simulink model "PH1_uGrid_ZC_carga"  (R2017a)
settings: Solver=ode4  StartTime=0.0  StopTime=6  FixedStep=1e-6  MaxStep=1e-4  RelTol=1e-3
InitFcn:
  | SimulinkInit
values from neighbouring files (symbols this model uses):
  J = 0.3    [SimulinkInit.m]
  K1 = 1.15    [SimulinkInit.m]
  K2 = 1    [SimulinkInit.m]
  K3 = 1    [SimulinkInit.m]
  P = 0.1    [SimulinkInit.m]
  Tao1 = 0.5    [SimulinkInit.m]
  Tao2 = 0.125    [SimulinkInit.m]
undefined symbols (not defined in the file or in its folder): G, GF, Ion, Lithium
libraries: powerlib x58, dsparch4 x12, powerlib_meascontrol x5, fl_lib x5, nesl_utility x4, mpclib x2, electricdrivelib x1, simulink x1
(part 2 of 2)

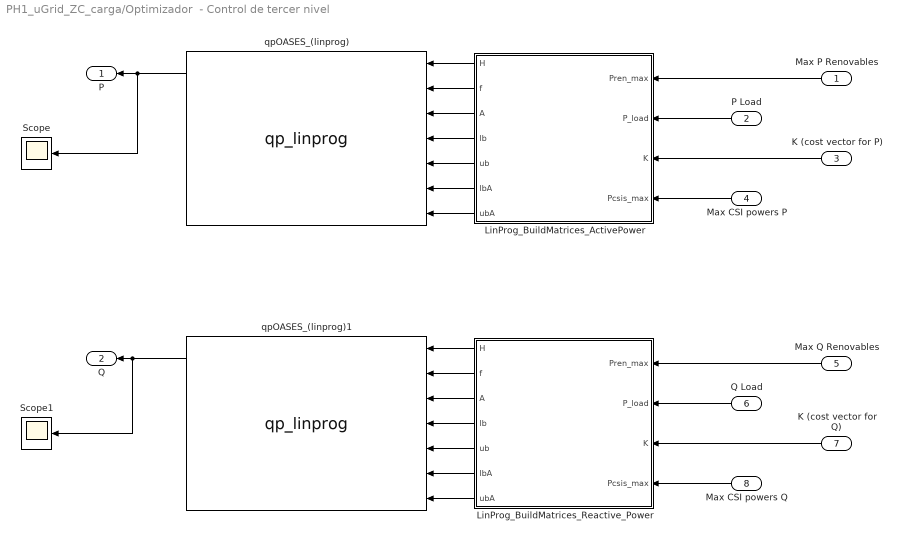
== system PH1_uGrid_ZC_carga/Optimizador  - Control de tercer nivel ==
  Max P Renovables : Inport
  P Load : Inport  Port=2
  K (cost vector for P) : Inport  Port=3
  Max CSI powers P : Inport  Port=4
  Max Q Renovables : Inport  Port=5
  Q Load : Inport  Port=6
  K (cost vector for Q) : Inport  Port=7
  Max CSI powers Q : Inport  Port=8
  LinProg_BuildMatrices_ActivePower : MATLAB Function  TreatAsAtomicUnit=on
  LinProg_BuildMatrices_Reactive_Power : MATLAB Function  TreatAsAtomicUnit=on
  Scope : Scope
  Scope1 : Scope
  qpOASES_(linprog) : S-Function  FunctionName=qp_linprog  SFunctionDeploymentMode=off  EnableBusSupport=off
  qpOASES_(linprog)1 : S-Function  FunctionName=qp_linprog  SFunctionDeploymentMode=off  EnableBusSupport=off
  P : Outport
  Q : Outport  Port=2
  wires:
  Max CSI powers P/1 -> LinProg_BuildMatrices_ActivePower/4(Pcsis_max)
  Max P Renovables/1 -> LinProg_BuildMatrices_ActivePower/1(Pren_max)
  LinProg_BuildMatrices_ActivePower/6(lbA) -> qpOASES_(linprog)/6
  LinProg_BuildMatrices_ActivePower/5(ub) -> qpOASES_(linprog)/5
  LinProg_BuildMatrices_ActivePower/7(ubA) -> qpOASES_(linprog)/7
  LinProg_BuildMatrices_ActivePower/2(f) -> qpOASES_(linprog)/2
  LinProg_BuildMatrices_ActivePower/4(lb) -> qpOASES_(linprog)/4
  LinProg_BuildMatrices_ActivePower/1(H) -> qpOASES_(linprog)/1
  K (cost vector for P)/1 -> LinProg_BuildMatrices_ActivePower/3(K)
  P Load/1 -> LinProg_BuildMatrices_ActivePower/2(P_load)
  LinProg_BuildMatrices_ActivePower/3(A) -> qpOASES_(linprog)/3
  LinProg_BuildMatrices_Reactive_Power/1(H) -> qpOASES_(linprog)1/1
  LinProg_BuildMatrices_Reactive_Power/5(ub) -> qpOASES_(linprog)1/5
  LinProg_BuildMatrices_Reactive_Power/3(A) -> qpOASES_(linprog)1/3
  LinProg_BuildMatrices_Reactive_Power/4(lb) -> qpOASES_(linprog)1/4
  LinProg_BuildMatrices_Reactive_Power/6(lbA) -> qpOASES_(linprog)1/6
  LinProg_BuildMatrices_Reactive_Power/2(f) -> qpOASES_(linprog)1/2
  LinProg_BuildMatrices_Reactive_Power/7(ubA) -> qpOASES_(linprog)1/7
  qpOASES_(linprog)/1 -> Scope/1, P/1
  qpOASES_(linprog)1/1 -> Scope1/1, Q/1
  Q Load/1 -> LinProg_BuildMatrices_Reactive_Power/2(P_load)
  K (cost vector for Q)/1 -> LinProg_BuildMatrices_Reactive_Power/3(K)
  Max Q Renovables/1 -> LinProg_BuildMatrices_Reactive_Power/1(Pren_max)
  Max CSI powers Q/1 -> LinProg_BuildMatrices_Reactive_Power/4(Pcsis_max)

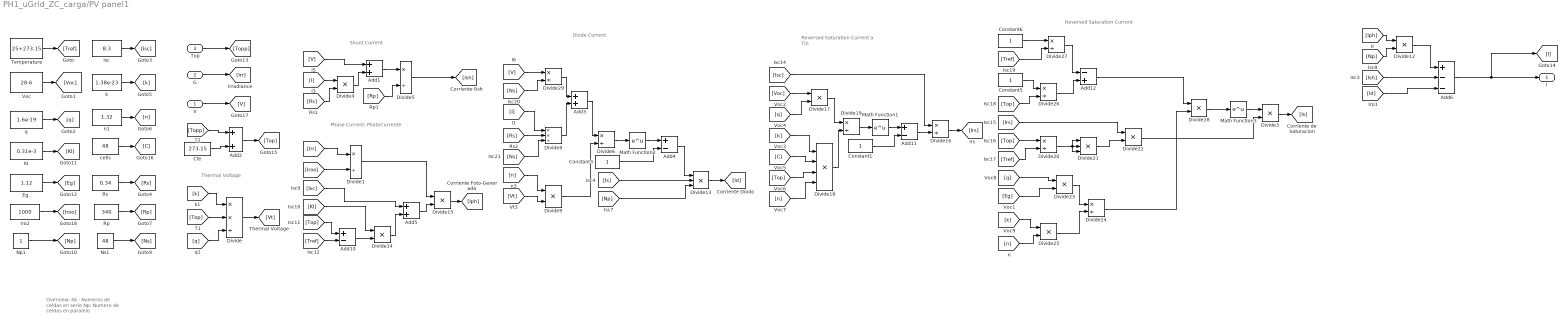
== system PH1_uGrid_ZC_carga/PV panel1 ==
  note: Overview:
      | Ns : Numeros de celdas en serie
      | Np: Numero de celdas en paralelo
  note: Thermal Voltage
  note: Shunt Current
  note: Phase Current- PhotoCurrente
  note: Diode Current
  note: Reversed Saturation Current a Tin
  note: Reversed Saturation Current
  V : Inport
  G : Inport  Port=2
  Top : Inport  Port=3
  Add{1..3,5} (4 alike) : Sum
  Add10 : Sum  Inputs=+-
  Add11 : Sum  Inputs=+-
  Add12 : Sum  Inputs=-+
  Add4 : Sum  Inputs=+-
  Add6 : Sum  Inputs=+--
  Constant{1,3,5..6} (4 alike) : Constant
  Cte : Constant  Value=273.15
  Divide : Product  Inputs=**/
  Divide{1,5..6,16,19..20,24,26..27,29} (10 alike) : Product  Inputs=*/
  Divide{3..4,9,12,14..15,17,22..23,25,28} (11 alike) : Product  Inputs=**
  Divide13 : Product  Inputs=***
  Divide18 : Product  Inputs=****
  Divide21 : Product  Inputs=***
  Divide8 : Product  Inputs=**/
  Eg. : Constant  Value=1.12
  Iro2 : Constant  Value=1000
  Isc : Constant  Value=8.3
  KI : Constant  Value=0.31e-3
  Math Function1 : Math  SaturateOnIntegerOverflow=on
  Math Function2 : Math  SaturateOnIntegerOverflow=on
  Math Function3 : Math  SaturateOnIntegerOverflow=on
  Np1 : Constant
  Ns1 : Constant  Value=48
  Rp : Constant  Value=340
  Rs : Constant  Value=0.34
  Temperature : Constant  Value=25+273.15
  Voc : Constant  Value=28.6
  cells : Constant  Value=48
  k : Constant  Value=1.38e-23
  n1 : Constant  Value=1.32
  q : Constant  Value=1.6e-19
  I : Outport
  wires:
  Temperature/1 -> [Tref]
  Voc/1 -> [Voc]
  q/1 -> [q]
  Isc/1 -> [Isc]
  k/1 -> [k]
  n1/1 -> [n]
  [k] -> Divide/1
  [Top] -> Divide/2
  [q] -> Divide/3
  Divide/1 -> [Vt]
  Divide3/1 -> [Is]
  [Ish] -> Add6/2
  Add6/1 -> I/1, [I]
  [I] -> Divide8/1
  [Rs] -> Divide8/2
  Divide8/1 -> Add3/2
  [n] -> Divide9/1
  [Vt] -> Divide9/2
  Divide9/1 -> Divide6/2
  Add3/1 -> Divide6/1
  Divide6/1 -> Math Function2/1
  Math Function2/1 -> Add4/1
  Add4/1 -> Divide13/1
  [Is] -> Divide13/2
  Divide13/1 -> [Id]
  Divide4/1 -> Add1/2
  Add1/1 -> Divide5/1
  [Rp] -> Divide5/2
  Divide5/1 -> [Ish]
  [Rs] -> Divide4/2
  [I] -> Divide4/1
  KI/1 -> [KI]
  Eg./1 -> [Eg]
  [V] -> Add1/1
  [Np] -> Divide13/3
  [Iph] -> Divide12/1
  [Np] -> Divide12/2
  Divide12/1 -> Add6/1
  [Isc] -> Add5/1
  [Top] -> Add10/1
  [Tref] -> Add10/2
  Add10/1 -> Divide14/2
  [KI] -> Divide14/1
  [Voc] -> Divide17/1
  [q] -> Divide17/2
  [k] -> Divide18/1
  [C] -> Divide18/2
  [Top] -> Divide18/3
  [n] -> Divide18/4
  Divide17/1 -> Divide19/1
  Divide18/1 -> Divide19/2
  Divide19/1 -> Math Function1/1
  Constant1/1 -> Add11/2
  Math Function1/1 -> Add11/1
  Add11/1 -> Divide16/2
  Divide16/1 -> [Irs]
  [Tref] -> Divide20/2
  [Top] -> Divide20/1
  Divide20/1 -> Divide21/2, Divide21/1, Divide21/3
  Divide21/1 -> Divide22/2
  [Irs] -> Divide22/1
  [q] -> Divide23/1
  Divide23/1 -> Divide24/1
  [k] -> Divide25/1
  [n] -> Divide25/2
  Divide25/1 -> Divide24/2
  Constant5/1 -> Divide26/1
  [Top] -> Divide26/2
  Constant6/1 -> Divide27/1
  [Tref] -> Divide27/2
  Divide27/1 -> Add12/1
  Divide26/1 -> Add12/2
  Add12/1 -> Divide28/1
  Divide24/1 -> Divide28/2
  Divide28/1 -> Math Function3/1
  Divide29/1 -> Add3/1
  [Ns] -> Divide29/2
  [V] -> Divide29/1
  [Ns] -> Divide8/3
  Divide14/1 -> Add5/2
  Add5/1 -> Divide15/2
  Divide15/1 -> [Iph]
  V/1 -> [V]
  G/1 -> [Irr]
  Top/1 -> [Topp]
  cells/1 -> [C]
  [Id] -> Add6/3
  Cte/1 -> Add2/2
  Add2/1 -> [Top]
  [Topp] -> Add2/1
  [Irr] -> Divide1/1
  [Iroo] -> Divide1/2
  Divide1/1 -> Divide15/1
  Iro2/1 -> [Iroo]
  Rs/1 -> [Rs]
  Rp/1 -> [Rp]
  Ns1/1 -> [Ns]
  Np1/1 -> [Np]
  Constant3/1 -> Add4/2
  [Isc] -> Divide16/1
  Math Function3/1 -> Divide3/1
  Divide22/1 -> Divide3/2
  [Eg] -> Divide23/2

== system PH1_uGrid_ZC_carga/Subsystem ==
  In1 : Inport
  Controlled Current Source : fl_lib/Electrical/Electrical Sources/Controlled Current Source
  Current Sensor : fl_lib/Electrical/Electrical Sensors/Current Sensor
  Electrical Reference : fl_lib/Electrical/Electrical Elements/Electrical Reference
  Id1 : Display
  Id3 : Display
  PS-Simulink Converter : nesl_utility/PS-Simulink Converter  PhysicalDomain=network_engine_domain  SubClassName=ps_output  LeftPortType=input  RightPortType=output  PseudoPeriodic=off  Frequencies=[]  Unit=1  AffineConversion=off
  PS-Simulink Converter1 : nesl_utility/PS-Simulink Converter  PhysicalDomain=network_engine_domain  SubClassName=ps_output  LeftPortType=input  RightPortType=output  PseudoPeriodic=off  Frequencies=[]  Unit=1  AffineConversion=off
  Resistor : fl_lib/Electrical/Electrical Elements/Resistor  R=10.02 Ohm  i_specify=off  i_priority=High  i=0 A  i_nominal_specify=off  i_nominal_unit=A  i_nominal_value=1  v_specify=off  v_priority=High  v=0 V  v_nominal_specify=off  v_nominal_unit=V  v_nominal_value=1
  Simulink-PS Converter1 : nesl_utility/Simulink-PS Converter  PhysicalDomain=network_engine_domain  SubClassName=ps_input  LeftPortType=input  RightPortType=output  PseudoPeriodic=off  Frequencies=[]  NoiseDistribution=none  NoiseParameters=[]  Unit=1  AffineConversion=off  FilteringAndDerivatives=zero  SimscapeFilterOrder=1  InputFilterTimeConstant=.000001  UdotUserProvided=0
  Solver Configuration : nesl_utility/Solver Configuration  PhysicalDomain=network_engine_domain  SubClassName=solver  LeftPortType=input  RightPortType=generic  Accelerate=off  Tones=[]  Harmonics=[]  SimulateNoise=off  Profile=off  UseLocalSampling=off  EnableSwitchedLinearOptims=on  FrequencyDomain=off  UseCCode=off  RelTol=0.001  AbsTol=1e-06  MinStep=1e-09  ToWorkspace=off  RevertToSquareIcSolve=off  NumHomotopyIterations=100  PhasorMode=off  PhasorModeNumHarmonics=1  OverrideAbsTol=off  DoDC=on  ResidualTolerance=1e-8  UseLocalSolver=on  LocalSolverChoice=NE_BACKWARD_EULER_ADVANCER  LocalSolverSampleTime=.1  DoFixedCost=off  MaxNonlinIter=8  MaxModeIter=2  LinearAlgebra=Sparse  DelaysMemoryBudget=1024  AutomaticFiltering=on  FilteringTimeConstant=0.001
  Voltage Sensor : fl_lib/Electrical/Electrical Sensors/Voltage Sensor
  V1 : Outport
  I : Outport  Port=2
  wires:
  PS-Simulink Converter1/1 -> I/1, Id1/1
  PS-Simulink Converter/1 -> V1/1, Id3/1
  In1/1 -> Simulink-PS Converter1/1
  connections:
  Voltage Sensor/RConn1 -- PS-Simulink Converter/LConn1
  Current Sensor/RConn2 -- Voltage Sensor/LConn1 -- Resistor/LConn1
  Controlled Current Source/RConn1 -- Simulink-PS Converter1/RConn1
  Electrical Reference/LConn1 -- Voltage Sensor/RConn2 -- Resistor/RConn1 -- Controlled Current Source/RConn2
  Current Sensor/RConn1 -- PS-Simulink Converter1/LConn1
  Controlled Current Source/LConn1 -- Current Sensor/LConn1 -- Solver Configuration/RConn1

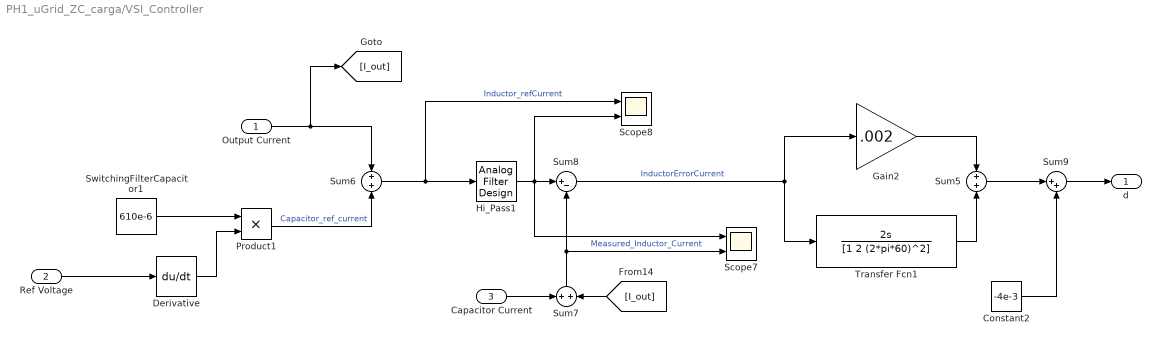
== system PH1_uGrid_ZC_carga/VSI_Controller ==
  Output Current : Inport
  Ref Voltage : Inport  Port=2
  Capacitor Current : Inport  Port=3
  Constant2 : Constant  Value=-4e-3
  Derivative : Derivative  CoefficientInTFapproximation=1e-3
  Gain2 : Gain  Gain=.002
  Hi_Pass1 : dsparch4/Analog Filter Design  method=Bessel  filttype=Highpass  N=1  Wlo=1*2*pi  Whi=80  Rp=2  Rs=40
  Product1 : Product
  Scope7 : Scope  NumInputPorts=2
  Scope8 : Scope  NumInputPorts=2
  Sum5 : Sum  Inputs=+|+
  Sum6 : Sum  Inputs=+|+
  Sum7 : Sum  Inputs=+|+
  Sum8 : Sum  Inputs=|+-
  Sum9 : Sum  Inputs=|++
  SwitchingFilterCapacitor1 : Constant  Value=610e-6
  Transfer Fcn1 : TransferFcn  Numerator=[2 0]  Denominator=[1 2 (2*pi*60)^2]
  d : Outport
  wires:
  Derivative/1 -> Product1/2
  Sum6/1 -> Hi_Pass1/1, Scope8/1  "Inductor_refCurrent"
  Sum8/1 -> Transfer Fcn1/1, Gain2/1  "InductorErrorCurrent"
  Ref Voltage/1 -> Derivative/1
  Constant2/1 -> Sum9/2
  Capacitor Current/1 -> Sum7/1
  Transfer Fcn1/1 -> Sum5/2
  Output Current/1 -> Sum6/1, [I_out]
  [I_out] -> Sum7/2
  Gain2/1 -> Sum5/1
  SwitchingFilterCapacitor1/1 -> Product1/1
  Hi_Pass1/1 -> Scope8/2, Sum8/1, Scope7/1
  Product1/1 -> Sum6/2  "Capacitor_ref_current"
  Sum9/1 -> d/1
  Sum5/1 -> Sum9/1
  Sum7/1 -> Scope7/2, Sum8/2  "Measured_Inductor_Current"

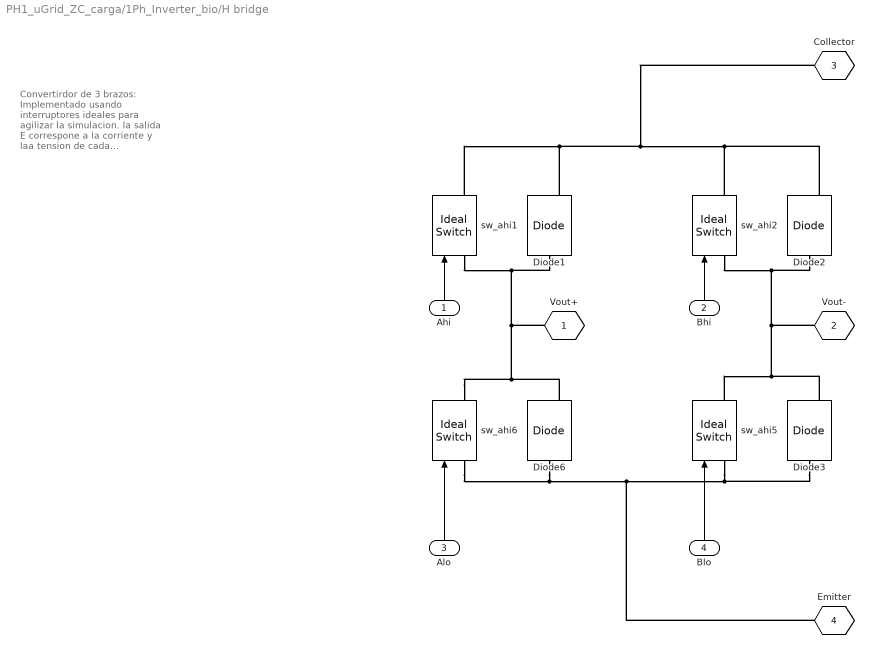
== system PH1_uGrid_ZC_carga/1Ph_Inverter_bio/H bridge ==
  note: Convertirdor de 3 brazos:
      |
      | Implementado usando interruptores
      | ideales para agilizar la simulacion.
      | la salida E correspone a la corriente y laa
      | tension de cada componente
      | (sea interruptor o diodo) y su respectiva
      | corriente. no tienen puerto de salida ya que no
      | son relevantes para lo que se desea simular.
      |
      | si g=0 interruptor no conduce.
      | si g=1 interruptor conduce.
      |
      | conmutacion ocurre instantaneamente sin
      | retardo.
  Ahi : Inport
  Bhi : Inport  Port=2
  Alo : Inport  Port=3
  Blo : Inport  Port=4
   sw_ahi{1..2,5..6} (4 alike) : powerlib/Power Electronics/Ideal Switch  Ron=0.1  Lon=0  IC=0  Rs=1e6  Cs=10e-12  Measurements=on
  Diode{1..3,6} (4 alike) : powerlib/Power Electronics/Diode  Ron=.2  Lon=0  Vf=0.8  IC=0  UseSnubber=0  Rs=0  Cs=0  Measurements=on
  " Vout+" : PMIOPort  Tag=PMCPort  Port=1  Side=Right
  Vout- : PMIOPort  Tag=PMCPort  Port=2  Side=Right
  Collector : PMIOPort  Tag=PMCPort  Port=3  Side=Right
  Emitter : PMIOPort  Tag=PMCPort  Port=4  Side=Right
  wires:
  Alo/1 -> " sw_ahi6"/1
  Ahi/1 -> " sw_ahi1"/1
  Blo/1 -> " sw_ahi5"/1
  Bhi/1 -> " sw_ahi2"/1
  connections:
  Diode3/RConn1 -- Vout-/RConn1 -- " sw_ahi2"/LConn1 -- Diode2/LConn1 -- " sw_ahi5"/RConn1
  Diode3/LConn1 -- Emitter/RConn1 -- Diode6/LConn1 -- " sw_ahi6"/LConn1 -- " sw_ahi5"/LConn1
  Diode2/RConn1 -- Collector/RConn1 -- " sw_ahi1"/RConn1 -- Diode1/RConn1 -- " sw_ahi2"/RConn1
  " sw_ahi6"/RConn1 -- Diode6/RConn1 -- " Vout+"/RConn1 -- Diode1/LConn1 -- " sw_ahi1"/LConn1

== system PH1_uGrid_ZC_carga/1Ph_Inverter_bio/Steper1 ==
  In1 : Inport
  Product : Product
  Step : Step  Time=st_time  SampleTime=samp_f
  Out1 : Outport
  wires:
  Step/1 -> Product/2
  In1/1 -> Product/1
  Product/1 -> Out1/1

== system PH1_uGrid_ZC_carga/1Ph_Inverter_bio/Steper3 ==
  In1 : Inport
  Product : Product
  Step : Step  Time=st_time  SampleTime=samp_f
  Out1 : Outport
  wires:
  Product/1 -> Out1/1
  In1/1 -> Product/1
  Step/1 -> Product/2

== system PH1_uGrid_ZC_carga/1Ph_Inverter_bio1/H bridge ==
  note: Convertirdor de 3 brazos:
      |
      | Implementado usando interruptores
      | ideales para agilizar la simulacion.
      | la salida E correspone a la corriente y laa
      | tension de cada componente
      | (sea interruptor o diodo) y su respectiva
      | corriente. no tienen puerto de salida ya que no
      | son relevantes para lo que se desea simular.
      |
      | si g=0 interruptor no conduce.
      | si g=1 interruptor conduce.
      |
      | conmutacion ocurre instantaneamente sin
      | retardo.
  Ahi : Inport
  Bhi : Inport  Port=2
  Alo : Inport  Port=3
  Blo : Inport  Port=4
   sw_ahi{1..2,5..6} (4 alike) : powerlib/Power Electronics/Ideal Switch  Ron=0.1  Lon=0  IC=0  Rs=1e6  Cs=10e-12  Measurements=on
  Diode{1..3,6} (4 alike) : powerlib/Power Electronics/Diode  Ron=.2  Lon=0  Vf=0.8  IC=0  UseSnubber=0  Rs=0  Cs=0  Measurements=on
  " Vout+" : PMIOPort  Tag=PMCPort  Port=1  Side=Right
  Vout- : PMIOPort  Tag=PMCPort  Port=2  Side=Right
  Collector : PMIOPort  Tag=PMCPort  Port=3  Side=Right
  Emitter : PMIOPort  Tag=PMCPort  Port=4  Side=Right
  wires:
  Alo/1 -> " sw_ahi6"/1
  Ahi/1 -> " sw_ahi1"/1
  Blo/1 -> " sw_ahi5"/1
  Bhi/1 -> " sw_ahi2"/1
  connections:
  Diode3/RConn1 -- Vout-/RConn1 -- " sw_ahi2"/LConn1 -- Diode2/LConn1 -- " sw_ahi5"/RConn1
  Diode3/LConn1 -- Emitter/RConn1 -- Diode6/LConn1 -- " sw_ahi6"/LConn1 -- " sw_ahi5"/LConn1
  Diode2/RConn1 -- Collector/RConn1 -- " sw_ahi1"/RConn1 -- Diode1/RConn1 -- " sw_ahi2"/RConn1
  " sw_ahi6"/RConn1 -- Diode6/RConn1 -- " Vout+"/RConn1 -- Diode1/LConn1 -- " sw_ahi1"/LConn1

== system PH1_uGrid_ZC_carga/1Ph_Inverter_bio1/Steper1 ==
  In1 : Inport
  Product : Product
  Step : Step  Time=st_time  SampleTime=samp_f
  Out1 : Outport
  wires:
  Step/1 -> Product/2
  In1/1 -> Product/1
  Product/1 -> Out1/1

== system PH1_uGrid_ZC_carga/1Ph_Inverter_bio1/Steper3 ==
  In1 : Inport
  Product : Product
  Step : Step  Time=st_time  SampleTime=samp_f
  Out1 : Outport
  wires:
  Product/1 -> Out1/1
  In1/1 -> Product/1
  Step/1 -> Product/2

== system PH1_uGrid_ZC_carga/1Ph_Inverter_diesel/H bridge ==
  note: Convertirdor de 3 brazos:
      |
      | Implementado usando interruptores
      | ideales para agilizar la simulacion.
      | la salida E correspone a la corriente y laa
      | tension de cada componente
      | (sea interruptor o diodo) y su respectiva
      | corriente. no tienen puerto de salida ya que no
      | son relevantes para lo que se desea simular.
      |
      | si g=0 interruptor no conduce.
      | si g=1 interruptor conduce.
      |
      | conmutacion ocurre instantaneamente sin
      | retardo.
  Ahi : Inport
  Bhi : Inport  Port=2
  Alo : Inport  Port=3
  Blo : Inport  Port=4
   sw_ahi{1..2,5..6} (4 alike) : powerlib/Power Electronics/Ideal Switch  Ron=0.1  Lon=0  IC=0  Rs=1e6  Cs=10e-12  Measurements=on
  Diode{1..3,6} (4 alike) : powerlib/Power Electronics/Diode  Ron=.2  Lon=0  Vf=0.8  IC=0  UseSnubber=0  Rs=0  Cs=0  Measurements=on
  " Vout+" : PMIOPort  Tag=PMCPort  Port=1  Side=Right
  Vout- : PMIOPort  Tag=PMCPort  Port=2  Side=Right
  Collector : PMIOPort  Tag=PMCPort  Port=3  Side=Right
  Emitter : PMIOPort  Tag=PMCPort  Port=4  Side=Right
  wires:
  Bhi/1 -> " sw_ahi2"/1
  Blo/1 -> " sw_ahi5"/1
  Ahi/1 -> " sw_ahi1"/1
  Alo/1 -> " sw_ahi6"/1
  connections:
  " sw_ahi1"/LConn1 -- Diode1/LConn1 -- " Vout+"/RConn1 -- Diode6/RConn1 -- " sw_ahi6"/RConn1
  " sw_ahi2"/RConn1 -- Diode1/RConn1 -- " sw_ahi1"/RConn1 -- Collector/RConn1 -- Diode2/RConn1
  " sw_ahi5"/LConn1 -- " sw_ahi6"/LConn1 -- Diode6/LConn1 -- Emitter/RConn1 -- Diode3/LConn1
  " sw_ahi5"/RConn1 -- Diode2/LConn1 -- " sw_ahi2"/LConn1 -- Vout-/RConn1 -- Diode3/RConn1

== system PH1_uGrid_ZC_carga/1Ph_Inverter_diesel/Steper1 ==
  In1 : Inport
  Product : Product
  Step : Step  Time=st_time  SampleTime=samp_f
  Out1 : Outport
  wires:
  Product/1 -> Out1/1
  In1/1 -> Product/1
  Step/1 -> Product/2

== system PH1_uGrid_ZC_carga/1Ph_Inverter_diesel/Steper3 ==
  In1 : Inport
  Product : Product
  Step : Step  Time=st_time  SampleTime=samp_f
  Out1 : Outport
  wires:
  Step/1 -> Product/2
  In1/1 -> Product/1
  Product/1 -> Out1/1

== system PH1_uGrid_ZC_carga/CSI_Control_BIO/Death_time ==
  In1 : Inport
  Product : Product
  Step : Step  Time=st_time  SampleTime=T
  Out1 : Outport
  wires:
  Product/1 -> Out1/1
  In1/1 -> Product/1
  Step/1 -> Product/2

== system PH1_uGrid_ZC_carga/CSI_Control_BIO/PR Controller_0_ref 1 ==
  ref : Inport
  real : Inport  Port=2
  K1 : Gain  Gain=Kp
  K2 : Gain  Gain=Ki
  Steper6 : Subsystem
  Sum : Sum  Inputs=+-
  Sum1 : Sum  Inputs=+|+
  Transfer Fcn : TransferFcn  Numerator=[1 0]  Denominator=[1 wa (w0)^2]
  Out1 : Outport
  wires:
  real/1 -> Sum/2
  ref/1 -> Sum/1
  Sum/1 -> Steper6/1(In1)
  K1/1 -> Sum1/1
  Transfer Fcn/1 -> Sum1/2
  K2/1 -> Transfer Fcn/1
  Steper6/1(Out1) -> K1/1, K2/1
  Sum1/1 -> Out1/1

== system PH1_uGrid_ZC_carga/CSI_Control_DIESEL/Death_time ==
  In1 : Inport
  Product : Product
  Step : Step  Time=st_time  SampleTime=T
  Out1 : Outport
  wires:
  Step/1 -> Product/2
  In1/1 -> Product/1
  Product/1 -> Out1/1

== system PH1_uGrid_ZC_carga/CSI_Control_DIESEL/PR Controller_0_ref 1 ==
  ref : Inport
  real : Inport  Port=2
  K1 : Gain  Gain=Kp
  K2 : Gain  Gain=Ki
  Steper6 : Subsystem
  Sum : Sum  Inputs=+-
  Sum1 : Sum  Inputs=+|+
  Transfer Fcn : TransferFcn  Numerator=[1 0]  Denominator=[1 wa (w0)^2]
  Out1 : Outport
  wires:
  Sum1/1 -> Out1/1
  Steper6/1(Out1) -> K2/1, K1/1
  K2/1 -> Transfer Fcn/1
  Transfer Fcn/1 -> Sum1/2
  K1/1 -> Sum1/1
  Sum/1 -> Steper6/1(In1)
  ref/1 -> Sum/1
  real/1 -> Sum/2

== system PH1_uGrid_ZC_carga/CSI_Control_BIO/PR Controller_0_ref 1/Steper6 ==
  In1 : Inport
  Product : Product
  Step : Step  Time=st_time  SampleTime=0
  Out1 : Outport
  wires:
  Product/1 -> Out1/1
  In1/1 -> Product/1
  Step/1 -> Product/2

== system PH1_uGrid_ZC_carga/CSI_Control_DIESEL/PR Controller_0_ref 1/Steper6 ==
  In1 : Inport
  Product : Product
  Step : Step  Time=st_time  SampleTime=0
  Out1 : Outport
  wires:
  Step/1 -> Product/2
  In1/1 -> Product/1
  Product/1 -> Out1/1

== matlab function PH1_uGrid_ZC_carga/1Ph_Inverter_diesel/not_pwm ==
  data: u input; y output
function y = fcn(u)
%#codegen

if(u==0 || u<0)
    a=15;
else
    a=0;
end;

y = a;

== matlab function PH1_uGrid_ZC_carga/1Ph_Inverter_bio/not_pwm ==
  data: u input; y output
function y = fcn(u)
%#codegen

if(u==0 || u<0)
    a=15;
else
    a=0;
end;

y = a;

== matlab function PH1_uGrid_ZC_carga/CSI_Control_BIO/PQ_singlePhase ==
  data: va input; p output; vb input; ia input; ib input; q output
function [p, q] = fcn(va, vb, ia, ib)
% Esta funcion calcula la potencia activa y reactiva instantanea
% para el caso mnosofasico. En la revision de 2 papers he observado
% que una manera de extender la teoria de potencia al caso monofasico
% es asumiendo la tension o corriente de una fase como la componente
% alpha y hacer un desfase de 90 grados para obtener una version
% artificial de beta.

paux=va*ia+vb*ib;
if(paux > 20e4)
    paux = 20e4;
end
if(paux < -20e4)
    paux = -20e-4;
end

p = paux/2; % potencia activa instantanea

qaux = vb*ia-va*ib;

if(qaux>20e4)
    qaux=20e4;
end
if(qaux<-20e4)
    qaux=-20e4;
end

q = qaux/2; % potencia reactiva instantanea

== matlab function PH1_uGrid_ZC_carga/CSI_Control_DIESEL/PQ2Iab_PH1 ==
  data: Va input; Ia output; Vb input; p input; q input; Ib output
function [Ia, Ib] = fcn(Va, Vb, p, q)
%#codegen

% divide by zero protection
if(abs((Va^2+Vb^2))<=1000*eps(0))
    det = 1/eps(0);
else
    det = 1/(Va^2+Vb^2); % constante auxiliar
end;
%det = 1/(Va^2+Vb^2);

Mat = det*[Va Vb; Vb -Va];
Iab = Mat*[2*p;2*q];

Iaaux = Iab(1);
Ibaux = Iab(2);

ilim=1e3;

if(Iaaux>ilim)
    Iaaux=ilim;
end;
if(Iaaux<-ilim)
    Iaaux =-ilim;    
end;

if(isnan(Iaaux))
    Iaaux=0;
end;
%-----------------


if(Ibaux>ilim)
    Ibaux=ilim;
end;
if(Ibaux<-ilim)
    Ibaux =-ilim;    
end;

if(isnan(Ibaux))
    Ibaux=0;
end;
%-----------------


Ia = Iaaux;
Ib = Ibaux;

== matlab function PH1_uGrid_ZC_carga/CSI_Control_DIESEL/PQ_singlePhase ==
  data: va input; p output; vb input; ia input; ib input; q output
function [p, q] = fcn(va, vb, ia, ib)
% Esta funcion calcula la potencia activa y reactiva instantanea
% para el caso mnosofasico. En la revision de 2 papers he observado
% que una manera de extender la teoria de potencia al caso monofasico
% es asumiendo la tension o corriente de una fase como la componente
% alpha y hacer un desfase de 90 grados para obtener una version
% artificial de beta.

paux=va*ia+vb*ib;
if(paux > 20e4)
    paux = 20e4;
end
if(paux < -20e4)
    paux = -20e-4;
end

p = paux/2; % potencia activa instantanea

qaux = vb*ia-va*ib;

if(qaux>20e4)
    qaux=20e4;
end
if(qaux<-20e4)
    qaux=-20e4;
end

q = qaux/2; % potencia reactiva instantanea

== matlab function PH1_uGrid_ZC_carga/1Ph_Inverter_bio1/not_pwm ==
  data: u input; y output
function y = fcn(u)
%#codegen

if(u==0 || u<0)
    a=15;
else
    a=0;
end;

y = a;

== matlab function PH1_uGrid_ZC_carga/MATLAB Function ==
  data: SOC input; MaxP output; MaxQ output
function [MaxP, MaxQ] = fcn(SOC)


%  funcion que calcula la potencia maxima que puede suministrar las fuentes
%  renovables deacuerdo a la cantidad de carga que hay almancenada en la
%  bateria. esta va de 0 a 100%


% estoc valores que aparecen a continuacion se pusieron de manera
% arbitraria. corresponde a una persona con especialidad en la parte de
% potencia electrica determinar el verdadero algoritmo para hallar la
% potencia que deberia suministrar el nodo de energia renovable deacuerdo a
% la carga de la bateria.

MaxP = 0;
MaxQ = 0;

if( SOC >= 90 )
    MaxP = 500;
    MaxQ = 5000;
end

if( SOC <= 90 )
    MaxP = 200;
    MaxQ = 4000;
end

if( SOC <= 70 )
    MaxP = 100;
    MaxQ = 1000;
end

if( SOC <= 60 )
    MaxP = 50;
    MaxQ = 500;
end

== matlab function PH1_uGrid_ZC_carga/CSI_Control_BIO/PQ2Iab_PH1 ==
  data: Va input; Ia output; Vb input; p input; q input; Ib output
function [Ia, Ib] = fcn(Va, Vb, p, q)
%#codegen

% divide by zero protection
if(abs((Va^2+Vb^2))<=1000*eps(0))
    det = 1/eps(0);
else
    det = 1/(Va^2+Vb^2); % constante auxiliar
end;
%det = 1/(Va^2+Vb^2);

Mat = det*[Va Vb; Vb -Va];
Iab = Mat*[2*p;2*q];

Iaaux = Iab(1);
Ibaux = Iab(2);

ilim=1e3;

if(Iaaux>ilim)
    Iaaux=ilim;
end;
if(Iaaux<-ilim)
    Iaaux =-ilim;    
end;

if(isnan(Iaaux))
    Iaaux=0;
end;
%-----------------


if(Ibaux>ilim)
    Ibaux=ilim;
end;
if(Ibaux<-ilim)
    Ibaux =-ilim;    
end;

if(isnan(Ibaux))
    Ibaux=0;
end;
%-----------------


Ia = Iaaux;
Ib = Ibaux;

== matlab function PH1_uGrid_ZC_carga/Optimizador  - Control de tercer nivel/LinProg_BuildMatrices_ActivePower ==
  data: H output; Pren_max input; f output; P_load input; K input; A output; lb output; ub output; lbA output; ubA output; Pcsis_max input
function [H, f, A, lb, ub, lbA, ubA] = fcn(Pren_max, P_load, K, Pcsis_max)

% Pr_max es la potencia maxima que puede suministrar el nodo de energias
% renovables.

% P_load es la potencia que consume la carga. ambas potencias son un vector
% de 2 componentes donde la primera componenete es la potencia activa y la
% segunda componenete es la potencia reactiva.

% Kp y Kq corresponde a un vector con los costos de la energia activa y 
% reactiva respectivamente para cada uno de los convertidores, en este caso
% bio y diesel solamente pero pueden agregarse tantas fuentes como se
% desee.

% Pin_max Qin_max corresponde a un vector con los valores maximos de
% potencia activa y reactiva que pueden generar cada una de las otras 
% fuentes diferentes a energias alternativas.


% El bloque qpOASES_(linprog) es un bloque que resuelve el problema standar
% de optimizacion cuadratica :
% 1/2 x' H x + x' f
% sujeto a unas restricciones. la matriz H corresponde a la parte
% cuadratica del problema mientras que f corresponde a la parte lineal. es
% decir que haciendo H = matriz de zeros, es posible reutilizar el bloque
% para solucionar problemas de programacion lineal, que es justamente lo
% que se hace en esta parte del modelo.

% La presente matlab function tiene como tarea formar las matrices f
% y A de restricciones apropiadas para que el bloque de qp oases realice la
% funcione de programacion lineal.

Pm = sum(Pcsis_max); % potencia activa maxima que pueden entregar todas las fuentes (en este caso bio y diesel)


D = P_load - Pren_max; % diferencia entre la potencia que puede generar
% renovables con la que consume la carga.


     % % % % % % % % % % % % % % % % % % % % % % % % % % % % %  
    % Formacion de las entradas para la programacion lineal.  %
     % % % % % % % % % % % % % % % % % % % % % % % % % % % % %  
     
% parte cuadratica de la funcion de coste que se pone en zeros para
% transformarlo en un problema de programacion lineal.
H = zeros(1, length(K)^2);

% funcion de coste lineal.
f = K;

% matriz de restricciones.
% esta formada con la idea de definir que la suma de todas las potencias
% deben almenos cubrir la cantidad de energia activa y reactiva que no
% puede suministrar renovables.
A = ones(1, length(K));

lb = zeros(1, length(K)); % potencia minima que puede generar cada uno de los generadores.
ub = [Pcsis_max]; % potencia maxima que pueden generar cada uno de los generadores.

ubA = [Pm]; % tambien esta relacionado con la potencia min, es un
% requerimiento para el blque de programacion lineal.

% depenediendo la diferencia entre la potencia que pide la carga y la que
% pueden suministrar energias renovables entonces lbA debe establecerce de
% manera conveniente para que el problema de programacion lineal tenga
% solucion.

% restriccion limite inferior para la potencia activa
if(D > 0) % en caso de que renovables no baste para alimentar la carga...
    if(D >= Pm)
        vp = Pm;
    else
        vp = D(1);
    end
else % si renovables basta para alimentar la carga. es decir D = 0 ó negativo
    vp = 0;
end

lbA = vp;

== matlab function PH1_uGrid_ZC_carga/Optimizador  - Control de tercer nivel/LinProg_BuildMatrices_Reactive_Power ==
  data: H output; Pren_max input; f output; P_load input; K input; A output; lb output; ub output; lbA output; ubA output; Pcsis_max input
function [H, f, A, lb, ub, lbA, ubA] = fcn(Pren_max, P_load, K, Pcsis_max)

% Pr_max es la potencia maxima que puede suministrar el nodo de energias
% renovables.

% P_load es la potencia que consume la carga. ambas potencias son un vector
% de 2 componentes donde la primera componenete es la potencia activa y la
% segunda componenete es la potencia reactiva.

% Kp y Kq corresponde a un vector con los costos de la energia activa y 
% reactiva respectivamente para cada uno de los convertidores, en este caso
% bio y diesel solamente pero pueden agregarse tantas fuentes como se
% desee.

% Pin_max Qin_max corresponde a un vector con los valores maximos de
% potencia activa y reactiva que pueden generar cada una de las otras 
% fuentes diferentes a energias alternativas.


% El bloque qpOASES_(linprog) es un bloque que resuelve el problema standar
% de optimizacion cuadratica :
% 1/2 x' H x + x' f
% sujeto a unas restricciones. la matriz H corresponde a la parte
% cuadratica del problema mientras que f corresponde a la parte lineal. es
% decir que haciendo H = matriz de zeros, es posible reutilizar el bloque
% para solucionar problemas de programacion lineal, que es justamente lo
% que se hace en esta parte del modelo.

% La presente matlab function tiene como tarea formar las matrices f
% y A de restricciones apropiadas para que el bloque de qp oases realice la
% funcione de programacion lineal.

Pm = sum(Pcsis_max); % potencia activa maxima que pueden entregar todas las fuentes (en este caso bio y diesel)


D = P_load - Pren_max; % diferencia entre la potencia que puede generar
% renovables con la que consume la carga.


     % % % % % % % % % % % % % % % % % % % % % % % % % % % % %  
    % Formacion de las entradas para la programacion lineal.  %
     % % % % % % % % % % % % % % % % % % % % % % % % % % % % %  
     
% parte cuadratica de la funcion de coste que se pone en zeros para
% transformarlo en un problema de programacion lineal.
H = zeros(1, length(K)^2);

% funcion de coste lineal.
f = K;

% matriz de restricciones.
% esta formada con la idea de definir que la suma de todas las potencias
% deben almenos cubrir la cantidad de energia activa y reactiva que no
% puede suministrar renovables.
A = ones(1, length(K));

lb = zeros(1, length(K)); % potencia minima que puede generar cada uno de los generadores.
ub = [Pcsis_max]; % potencia maxima que pueden generar cada uno de los generadores.

ubA = [Pm]; % tambien esta relacionado con la potencia min, es un
% requerimiento para el blque de programacion lineal.

% depenediendo la diferencia entre la potencia que pide la carga y la que
% pueden suministrar energias renovables entonces lbA debe establecerce de
% manera conveniente para que el problema de programacion lineal tenga
% solucion.

% restriccion limite inferior para la potencia activa
if(D > 0) % en caso de que renovables no baste para alimentar la carga...
    if(D >= Pm)
        vp = Pm;
    else
        vp = D(1);
    end
else % si renovables basta para alimentar la carga. es decir D = 0 ó negativo
    vp = 0;
end

lbA = vp;

== matlab function PH1_uGrid_ZC_carga/MPC_bio/MPC_MatCalc ==
  data: ref input; PQ input; Hv output; F output; A output; lb output; ub output; lbA output; ubA output; Du input; MPCout input; G input; GF input
function [Hv, F, A, lb, ub, lbA, ubA] = MPC(ref, PQ, Du, MPCout, G, GF)

%%parametros del MPC


p = 100; % horizonte de prediccion
Nu = 100; % horizonte de control


%% Calculo de la salida de control.

H = G'*G+eye(2*Nu)*3000; % parte cuadratica del qp

ym = [ ones(p, 1)*PQ(1); ones(p, 1)*PQ(2) ]; % vector de la medida de tempearatura actual.

w = [ ones(p, 1)*ref(1); ones(p, 1)*ref(2) ]; % vector señal setpoint.

L = GF*Du+ym; % respuesta libre.

F = 2*(L-w)'*G; % parte lineal del problema qp.

A = zeros(1, 4*Nu*Nu);

lbA = zeros(1, 2*Nu);

ubA = zeros(1, 2*Nu);

Hv = M2V(H);

hip = HiBound(MPCout(1), 600, 10);
hiq = HiBound(MPCout(2), 5000, 1000);

lop = LowBound(MPCout(1), -100, -10);
loq = LowBound(MPCout(2), -100, -1000);

lb = [ones(1, Nu)*lop ones(1, Nu)*loq];
ub = [ones(1, Nu)*hip ones(1, Nu)*hiq];
end

% el control mpc implementado halla mediante programacion cuadratica
% los delta de u optimos deacuerdo a la funcion de coste. por este motivo
% es necesario implementar una logica adicional que permita limitar
% los valores de u (la salida) ya que estos no se manupilan directamente
% en el problema de programacion cuadratica.

% esta logica se implementan en las dos funciones locales que se encuentran
% a continuacion. una funcion define el limite superior y otra funcion para
% definir el limite inferior de los deltas de u deacuerdo al valor actual
% de u para asegurar que tanto los deltas de u como el valor de u esten
% limitados.
% esta funcion solo es correcta si max y Dmax son valores positivos.
function y = HiBound(X, max, Dmax)
    if(X>=0) % si la potencia X es positiva:
        if(max >= X)% si X no ha superado la potencia maxima:
            if(max-X >= Dmax) % si la distancia supera el cambio maximo deseado
                r = Dmax;
            else % si es menor al cambio maximo deseado
                r = max-X;
            end
        else % si X supera la potencia maxima deseada
            r = 0; % el delta maximo es 0 para que no se incremente mas.
        end
    else % si la potencia X es negativa, el incremento maximo es
        r = Dmax;
    end
    y = r;
end

% esta funcion para el lower bound se penso para trbajar con valores
% negativos. si min y Dmin no es negativo la funcion no funciona
% correctamente.
function y = LowBound(X, minv, Dmin)
    if(X<=0) % si la potencia X esta en el cuadrante inferior:
        if(minv <= X)% si X es mayor que la potencia minima:
            if(minv-X <= Dmin) % si la distancia supera el cambio maximo deseado
                r = Dmin;
            else % si es mayor al cambio maximo deseado
                r = minv-X;
            end
        else % si X es menor la potencia maxima deseada
            r = 0; % el delta maximo es 0 para que no se decremente mas.
        end
    else % si la potencia X es positiva, el decremento maximo es
        r = Dmin;
    end
    y = r;
end

== matlab function PH1_uGrid_ZC_carga/MPC_bio/MPC_OutLogic ==
  data: MPCout output; duv input; Duv output
function [MPCout, Duv] = MPC_out_Logic(duv)

%%parametros del MPC
Nu = 100; % horizonte de control.


%% variables del MPC
persistent Du; % deltas de u 
persistent out; % salida actual del conrolador MPC.

if isempty(Du) % inicializacion de los deltas de uu
    Du = zeros(2*Nu, 1);
end

if isempty(out) % inicializaion de la salida del controlador MPC
    out = [0; 0];
end


du = [duv(1), duv(Nu+1)];


Du = [du(1); Du(1:Nu-1); du(2); Du(Nu+1:end-1)];% actualizar historial deltas de u.

out = [ out(1)+du(1); out(2)+du(2) ]; %calcular salida del controlador.

MPCout = out;
Duv = Du;

== matlab function PH1_uGrid_ZC_carga/MPC_bio1/MPC_MatCalc ==
  data: ref input; PQ input; Hv output; F output; A output; lb output; ub output; lbA output; ubA output; Du input; MPCout input; G input; GF input
function [Hv, F, A, lb, ub, lbA, ubA] = MPC(ref, PQ, Du, MPCout, G, GF)

%%parametros del MPC


p = 100; % horizonte de prediccion
Nu = 100; % horizonte de control


%% Calculo de la salida de control.

H = G'*G+eye(2*Nu)*3000; % parte cuadratica del qp

ym = [ ones(p, 1)*PQ(1); ones(p, 1)*PQ(2) ]; % vector de la medida de tempearatura actual.

w = [ ones(p, 1)*ref(1); ones(p, 1)*ref(2) ]; % vector señal setpoint.

L = GF*Du+ym; % respuesta libre.

F = 2*(L-w)'*G; % parte lineal del problema qp.

A = zeros(1, 4*Nu*Nu);

lbA = zeros(1, 2*Nu);

ubA = zeros(1, 2*Nu);

Hv = M2V(H);

hip = HiBound(MPCout(1), 600, 10);
hiq = HiBound(MPCout(2), 5000, 1000);

lop = LowBound(MPCout(1), -100, -10);
loq = LowBound(MPCout(2), -100, -1000);

lb = [ones(1, Nu)*lop ones(1, Nu)*loq];
ub = [ones(1, Nu)*hip ones(1, Nu)*hiq];
end

% el control mpc implementado halla mediante programacion cuadratica
% los delta de u optimos deacuerdo a la funcion de coste. por este motivo
% es necesario implementar una logica adicional que permita limitar
% los valores de u (la salida) ya que estos no se manupilan directamente
% en el problema de programacion cuadratica.

% esta logica se implementan en las dos funciones locales que se encuentran
% a continuacion. una funcion define el limite superior y otra funcion para
% definir el limite inferior de los deltas de u deacuerdo al valor actual
% de u para asegurar que tanto los deltas de u como el valor de u esten
% limitados.
% esta funcion solo es correcta si max y Dmax son valores positivos.
function y = HiBound(X, max, Dmax)
    if(X>=0) % si la potencia X es positiva:
        if(max >= X)% si X no ha superado la potencia maxima:
            if(max-X >= Dmax) % si la distancia supera el cambio maximo deseado
                r = Dmax;
            else % si es menor al cambio maximo deseado
                r = max-X;
            end
        else % si X supera la potencia maxima deseada
            r = 0; % el delta maximo es 0 para que no se incremente mas.
        end
    else % si la potencia X es negativa, el incremento maximo es
        r = Dmax;
    end
    y = r;
end

% esta funcion para el lower bound se penso para trbajar con valores
% negativos. si min y Dmin no es negativo la funcion no funciona
% correctamente.
function y = LowBound(X, minv, Dmin)
    if(X<=0) % si la potencia X esta en el cuadrante inferior:
        if(minv <= X)% si X es mayor que la potencia minima:
            if(minv-X <= Dmin) % si la distancia supera el cambio maximo deseado
                r = Dmin;
            else % si es mayor al cambio maximo deseado
                r = minv-X;
            end
        else % si X es menor la potencia maxima deseada
            r = 0; % el delta maximo es 0 para que no se decremente mas.
        end
    else % si la potencia X es positiva, el decremento maximo es
        r = Dmin;
    end
    y = r;
end

== matlab function PH1_uGrid_ZC_carga/MPC_bio1/MPC_OutLogic ==
  data: MPCout output; duv input; Duv output
function [MPCout, Duv] = MPC_out_Logic(duv)

%%parametros del MPC
Nu = 100; % horizonte de control.


%% variables del MPC
persistent Du; % deltas de u 
persistent out; % salida actual del conrolador MPC.

if isempty(Du) % inicializacion de los deltas de uu
    Du = zeros(2*Nu, 1);
end

if isempty(out) % inicializaion de la salida del controlador MPC
    out = [0; 0];
end


du = [duv(1), duv(Nu+1)];


Du = [du(1); Du(1:Nu-1); du(2); Du(Nu+1:end-1)];% actualizar historial deltas de u.

out = [ out(1)+du(1); out(2)+du(2) ]; %calcular salida del controlador.

MPCout = out;
Duv = Du;

== matlab function PH1_uGrid_ZC_carga/LinearProg Potencia Activa ==
  data: P_load input; Pbo output; P_e_alt input; kb input; kd input; PdMax input; PbMax input; Pdo output
function [Pbo, Pdo] = fcn(P_load, P_e_alt, kb, kd, PdMax, PbMax)%, P_e_alt_min)

% P_load es la potencia que se requiere en la carga.

% P_e_alt es la potencia estimada de generacion de las energias
% alternativas

% kb y kd son los pesos de las funcion de costo.

% las salidas son las potencias optimas para bio y diesel

Pb=0;
Pd=0;

D_P_e_alt = P_e_alt %- P_e_alt_min % superaavit de energia alternativa.

flagDelt = 0;

if(D_P_e_alt >= P_load)
    flagDelt = 1;
end
   

if(flagDelt==0)
    P_trad = P_load - D_P_e_alt;
    % flag: variable que indica si tiene sentido evaluar los
    % if's que se encuentran mas adelante. es decir, si flag = 0 
    % despues del primer if entonces NO se le esta pidiendo al sistema
    % mas potencia de la que puede generar y portante el problema de 
    % optimizacion lineal tiene sentido.
    % entonces 
    flag=0;

    if(P_trad>PdMax+PbMax)
        Pd=PdMax;
        Pb=PbMax;
        flag=1;
    end

    % si ambas energias tienen el mismo factor de costo.
    if(kd==kb && flag==0)
        Pb=P_trad/2;
        Pd=P_trad/2;
    end

    % si la energia diesel es mas cara que la biomasa.
    if(kd>kb && flag==0)
        if(P_trad<=PbMax)
            Pb=P_trad;
            Pd=0;
        else
            Pb=PbMax;
            Pd=P_trad-PbMax;
        end
    end

    % si la biomasa es mas cara que la diesel.
    if(kd<kb && flag==0)
        if(P_trad<=PdMax)
            Pd=P_trad;
            Pb=0;
        else
            Pd=PdMax;
            Pb=P_trad-PdMax;
        end
    end
end

Pbo=Pb;
Pdo=Pd;

== matlab function PH1_uGrid_ZC_carga/LinearProg Potenica Reactiva ==
  data: Q_load input; Qbo output; Q_e_alt input; kb input; kd input; QdMax input; QbMax input; Qdo output
function [Qbo, Qdo] = fcn(Q_load, Q_e_alt, kb, kd, QdMax, QbMax)

% Q_load es la potencia que se requiere en la carga.

% Q_e_alt es la potencia estimada de generacion de las energias
% alternativas

% kb y kd son los pesos de las funcion de costo.

% las salidas son las potencias optimas para bio y diesel

Qb=0;
Qd=0;

D_P_e_alt = Q_e_alt ;%- Q_e_alt_min % superaavit de energia alternativa.

flagDelt = 0;

if(D_P_e_alt >= Q_load)
    flagDelt = 1;
end
   

if(flagDelt==0)
    Q_trad = Q_load - D_P_e_alt;
    % flag: variable que indica si tiene sentido evaluar los
    % if's que se encuentran mas adelante. es decir, si flag = 0 
    % despues del primer if entonces NO se le esta pidiendo al sistema
    % mas potencia de la que puede generar y portante el problema de 
    % optimizacion lineal tiene sentido.
    % entonces 
    flag=0;

    if(Q_trad>QdMax+QbMax)
        Qd=QdMax;
        Qb=QbMax;
        flag=1;
    end

    % si ambas energias tienen el mismo factor de costo.
    if(kd==kb && flag==0)
        Qb=Q_trad/2;
        Qd=Q_trad/2;
    end

    % si la energia diesel es mas cara que la biomasa.
    if(kd>kb && flag==0)
        if(Q_trad<=QbMax)
            Qb=Q_trad;
            Qd=0;
        else
            Qb=QbMax;
            Qd=Q_trad-QbMax;
        end
    end

    % si la biomasa es mas cara que la diesel.
    if(kd<kb && flag==0)
        if(Q_trad<=QdMax)
            Qd=Q_trad;
            Qb=0;
        else
            Qd=QdMax;
            Qb=Q_trad-QdMax;
        end
    end
end

Qbo=Qb;
Qdo=Qd;

== matlab function PH1_uGrid_ZC_carga/MATLAB Function1 ==
  data: SOC input; MaxP output; MaxQ output
function [MaxP, MaxQ] = fcn(SOC)


%  funcion que calcula la potencia maxima que puede suministrar las fuentes
%  renovables deacuerdo a la cantidad de carga que hay almancenada en la
%  bateria. esta va de 0 a 100%


% estoc valores que aparecen a continuacion se pusieron de manera
% arbitraria. corresponde a una persona con especialidad en la parte de
% potencia electrica determinar el verdadero algoritmo para hallar la
% potencia que deberia suministrar el nodo de energia renovable deacuerdo a
% la carga de la bateria.

MaxP = 0;
MaxQ = 0;

if( SOC >= 90 )
    MaxP = 500;
    MaxQ = 5000;
end

if( SOC <= 90 )
    MaxP = 200;
    MaxQ = 4000;
end

if( SOC <= 70 )
    MaxP = 100;
    MaxQ = 1000;
end

if( SOC <= 60 )
    MaxP = 50;
    MaxQ = 500;
end
